simulink library "MedusaPremix"  (R2022b)
settings: Solver=VariableStepAuto  StartTime=0.0  StopTime=10.0  RelTol=1e-3
values from neighbouring files (symbols this model uses):
  PremixConfig = struct('sample_rate_in_hertz', sample_rate_in_hertz,                            'frame_size', frame_size,                            'rgain_SILENT_GAIN', rgain_SILENT_GAIN,                            'granularity', internal_granularity,                            'LR_in', LR_in, 'LR_out', LR_out,                            'CS_in', CS_in, 'CS_out', CS_out,                            'NumCenterOut' ...(+550 chars)    [MedusaPremixInit.m]
  PremixTune = MedusaPremixTuneInit(tuneFileName, headrestTuneFileName, overheadTuneFileName, MedusaParams)    [MedusaPremixInit.m]    (also in MedusaPremixTuneInit.m = load(tuneFileName))
undefined symbols (not defined in the file or in its folder): carModel, mode, MSConfig, Row
libraries: TuneVar x286, TOP x202, dspmtrx3 x146, FeaturePath x86, matrix_library x20, PooliirLib x8, Pooliir x4
(part 17 of 22)

== matlab function MedusaPremix/PremixWithMonoSurroundAndCae/SLC Tuning/Detent Level Right/Trivial Translation ==
  data: TOP output size=[MedusaPremixConfig.LR_out MedusaPremixConfig.LR_in]; detentGain_Right input; MedusaPremixConfig parameter; TOP_CAE output size=[MedusaPremixConfig.LR_out MedusaPremixConfig.NumTailComp.LR]
  events: trigger input FUNCTION_CALL_EVENT
function [TOP, TOP_CAE]  = fcn(detentGain_Right, MedusaPremixConfig)
%#codegen
numLRIn = MedusaPremixConfig.LR_in;
NumCAEWeights = MedusaPremixConfig.NumTailComp.LR;

NumRows = MedusaPremixConfig.LR_out;
NumColumns = numLRIn + NumCAEWeights;
if(~ MedusaPremixConfig.includeCAE)
    NumColumns = numLRIn;
end

% Checks if the parameter satisfies dimensionality requirements
if(detentGain_Right.Size(1) ~= NumRows || detentGain_Right.Size(2) ~= NumColumns)
    TranslateError('The parameter ''medusa_premix_right_detent'' must be a matrix consisting of %d rows and %d columns.', NumRows, NumColumns);
end

% Checks if the parameter values follow bound requirements
checkValues = (detentGain_Right.Value < 0);    
if(sum(sum(checkValues)))       % Results in 0 if all values in the matrix respect the bound requirements
    TranslateError('The weights in ''medusa_premix_right_detent'' must be greater than or equal to 0.');
end

% Assigning the parameter values to respective tuneTOPS
TOP = detentGain_Right.Value(:, 1:numLRIn);
if(~ MedusaPremixConfig.includeCAE)
    TOP_CAE = zeros(NumRows, NumCAEWeights);
else
    TOP_CAE = detentGain_Right.Value(:, numLRIn+1:end);
end

end

== matlab function MedusaPremix/PremixWithMonoSurroundAndCae/SLC Tuning/Interpolation Method/Trivial Translation ==
  data: TOP output; interpolationMethod input
  events: trigger input FUNCTION_CALL_EVENT
function TOP  = fcn(interpolationMethod)
%#codegen
% Checks if the parameter satisfies dimensionality requirements
if(numel(interpolationMethod.Value) ~= 1)
   TranslateError('The parameter ''medusa_surround_db_interpolation'' must be single dimensional.'); 
end

% Checks if the parameter value follows bound requirements
if((interpolationMethod.Value ~= 0) && (interpolationMethod.Value ~= 1))
   TranslateError('The value of ''medusa_surround_db_interpolation'' must be either 0 (for linear interpolation) or 1 (for dB-linear interpolation).'); 
end

TOP = interpolationMethod.Value;

end

== matlab function MedusaPremix/PremixWithMonoSurroundAndCae/SLC Tuning/Max Level CS/Trivial Translation ==
  data: TOP output size=[MedusaPremixConfig.CS_out MedusaPremixConfig.CS_in]; maxGain_CS input; MedusaPremixConfig parameter; TOP_CAE output size=[MedusaPremixConfig.CS_out MedusaPremixConfig.NumTailComp.CS]
  events: trigger input FUNCTION_CALL_EVENT
function [TOP, TOP_CAE] = fcn(maxGain_CS, MedusaPremixConfig)
%#codegen
numCSIn = MedusaPremixConfig.CS_in;
NumCAEWeights = MedusaPremixConfig.NumTailComp.CS;

NumRows = MedusaPremixConfig.CS_out;
NumColumns = numCSIn + NumCAEWeights;
if(~ MedusaPremixConfig.includeCAE)
    NumColumns = numCSIn;
end

% Checks if the parameter satisfies dimensionality requirements
if(maxGain_CS.Size(1) ~= NumRows || maxGain_CS.Size(2) ~= NumColumns)
    TranslateError('The parameter ''medusa_premix_cs_max'' must be a matrix consisting of %d rows and %d columns.', NumRows, NumColumns);
end

% Checks if the parameter values follow bound requirements
checkValues = (maxGain_CS.Value < 0);
if(sum(sum(checkValues)))          % Results in 0 if all values in the matrix respect the bound requirements
    TranslateError('The weights in ''medusa_premix_cs_max'' must be greater than or equal to 0.');
end

% Assigning the parameter values to respective tuneTOPS
TOP = maxGain_CS.Value(:, 1:numCSIn);
if(~ MedusaPremixConfig.includeCAE)
    TOP_CAE = zeros(NumRows, NumCAEWeights);
else
    TOP_CAE = maxGain_CS.Value(:, numCSIn+1:end);
end

end

== matlab function MedusaPremix/PremixWithMonoSurroundAndCae/SLC Tuning/Max Level Left/Trivial Translation ==
  data: TOP output size=[MedusaPremixConfig.LR_out MedusaPremixConfig.LR_in]; maxGain_Left input; MedusaPremixConfig parameter; TOP_CAE output size=[MedusaPremixConfig.LR_out MedusaPremixConfig.NumTailComp.LR]
  events: trigger input FUNCTION_CALL_EVENT
function [TOP, TOP_CAE]  = fcn(maxGain_Left, MedusaPremixConfig)
%#codegen
numLRIn = MedusaPremixConfig.LR_in;
NumCAEWeights = MedusaPremixConfig.NumTailComp.LR;

NumRows = MedusaPremixConfig.LR_out;
NumColumns = numLRIn + NumCAEWeights;
if(~ MedusaPremixConfig.includeCAE)
    NumColumns = numLRIn;
end

% Checks if the parameter satisfies dimensionality requirements
if(maxGain_Left.Size(1) ~= NumRows || maxGain_Left.Size(2) ~= NumColumns)
    TranslateError('The parameter ''medusa_premix_left_max'' must be a matrix consisting of %d rows and %d columns.', NumRows, NumColumns);
end

% Checks if the parameter values follow bound requirements
checkValues = (maxGain_Left.Value < 0);
if(sum(sum(checkValues)))          % Results in 0 if all values in the matrix respect the bound requirements
    TranslateError('The weights in ''medusa_premix_left_max'' must be greater than or equal to 0.');
end

% Assigning the parameter values to respective tuneTOPS
TOP = maxGain_Left.Value(:, 1:numLRIn);
if(~ MedusaPremixConfig.includeCAE)
    TOP_CAE = zeros(NumRows, NumCAEWeights);
else
    TOP_CAE = maxGain_Left.Value(:, numLRIn+1:end);
end

end

== matlab function MedusaPremix/PremixWithMonoSurroundAndCae/SLC Tuning/Max Level Right/Trivial Translation ==
  data: TOP output size=[MedusaPremixConfig.LR_out MedusaPremixConfig.LR_in]; maxGain_Right input; MedusaPremixConfig parameter; TOP_CAE output size=[MedusaPremixConfig.LR_out MedusaPremixConfig.NumTailComp.LR]
  events: trigger input FUNCTION_CALL_EVENT
function [TOP, TOP_CAE]  = fcn(maxGain_Right, MedusaPremixConfig)
%#codegen
numLRIn = MedusaPremixConfig.LR_in;
NumCAEWeights = MedusaPremixConfig.NumTailComp.LR;

NumRows = MedusaPremixConfig.LR_out;
NumColumns = numLRIn + NumCAEWeights;
if(~ MedusaPremixConfig.includeCAE)
    NumColumns = numLRIn;
end

% Checks if the parameter satisfies dimensionality requirements
if(maxGain_Right.Size(1) ~= NumRows || maxGain_Right.Size(2) ~= NumColumns)
    TranslateError('The parameter ''medusa_premix_right_max'' must be a matrix consisting of %d rows and %d columns.', NumRows, NumColumns);
end

% Checks if the parameter values follow bound requirements
checkValues = (maxGain_Right.Value < 0);
if(sum(sum(checkValues)))          % Results in 0 if all values in the matrix respect the bound requirements
    TranslateError('The weights in ''medusa_premix_right_max'' must be greater than or equal to 0.');
end

% Assigning the parameter values to respective tuneTOPS
TOP = maxGain_Right.Value(:, 1:numLRIn);
if(~ MedusaPremixConfig.includeCAE)
    TOP_CAE = zeros(NumRows, NumCAEWeights);
else
    TOP_CAE = maxGain_Right.Value(:, numLRIn+1:end);
end

end

== matlab function MedusaPremix/PremixWithMonoSurroundAndCae/SLC Tuning/Min Level CS/Trivial Translation ==
  data: TOP output size=[MedusaPremixConfig.CS_out MedusaPremixConfig.CS_in]; minGain_CS input; MedusaPremixConfig parameter; TOP_CAE output size=[MedusaPremixConfig.CS_out MedusaPremixConfig.NumTailComp.CS]
  events: trigger input FUNCTION_CALL_EVENT
function [TOP, TOP_CAE]  = fcn(minGain_CS, MedusaPremixConfig)
%#codegen
numCSIn = MedusaPremixConfig.CS_in;
NumCAEWeights = MedusaPremixConfig.NumTailComp.CS;

NumRows = MedusaPremixConfig.CS_out;
NumColumns = numCSIn + NumCAEWeights;
if(~ MedusaPremixConfig.includeCAE)
    NumColumns = numCSIn;
end

% Checks if the parameter satisfies dimensionality requirements
if(minGain_CS.Size(1) ~= NumRows || minGain_CS.Size(2) ~= NumColumns)
    TranslateError('The parameter ''medusa_premix_cs_min'' must be a matrix consisting of %d rows and %d columns.', NumRows, NumColumns);
end

% Checks if the parameter values follow bound requirements
checkValues = (minGain_CS.Value < 0);
if(sum(sum(checkValues)))          % Results in 0 if all values in the matrix respect the bound requirements
    TranslateError('The weights in ''medusa_premix_cs_min'' must be greater than or equal to 0.');
end

% Assigning the parameter values to respective tuneTOPS
TOP = minGain_CS.Value(:, 1:numCSIn);
if(~ MedusaPremixConfig.includeCAE)
    TOP_CAE = zeros(NumRows, NumCAEWeights);
else
    TOP_CAE = minGain_CS.Value(:, numCSIn+1:end);
end

end

== matlab function MedusaPremix/PremixWithMonoSurroundAndCae/SLC Tuning/Min Level Left/Trivial Translation ==
  data: TOP output size=[MedusaPremixConfig.LR_out MedusaPremixConfig.LR_in]; minGain_Left input; MedusaPremixConfig parameter; TOP_CAE output size=[MedusaPremixConfig.LR_out MedusaPremixConfig.NumTailComp.LR]
  events: trigger input FUNCTION_CALL_EVENT
function [TOP, TOP_CAE]  = fcn(minGain_Left, MedusaPremixConfig)
%#codegen
numLRIn = MedusaPremixConfig.LR_in;
NumCAEWeights = MedusaPremixConfig.NumTailComp.LR;

NumRows = MedusaPremixConfig.LR_out;
NumColumns = numLRIn + NumCAEWeights;
if(~ MedusaPremixConfig.includeCAE)
    NumColumns = numLRIn;
end

% Checks if the parameter satisfies dimensionality requirements
if(minGain_Left.Size(1) ~= NumRows || minGain_Left.Size(2) ~= NumColumns)
    TranslateError('The parameter ''medusa_premix_left_min'' must be a matrix consisting of %d rows and %d columns.', NumRows, NumColumns);
end

% Checks if the parameter values follow bound requirements
checkValues = (minGain_Left.Value < 0);
if(sum(sum(checkValues)))          % Results in 0 if all values in the matrix respect the bound requirements
    TranslateError('The weights in ''medusa_premix_left_min'' must be greater than or equal to 0.');
end

% Assigning the parameter values to respective tuneTOPS
TOP = minGain_Left.Value(:, 1:numLRIn);
if(~ MedusaPremixConfig.includeCAE)
    TOP_CAE = zeros(NumRows, NumCAEWeights);
else
    TOP_CAE = minGain_Left.Value(:, numLRIn+1:end);
end

end

== matlab function MedusaPremix/PremixWithMonoSurroundAndCae/SLC Tuning/Min Level Right/Trivial Translation ==
  data: TOP output size=[MedusaPremixConfig.LR_out MedusaPremixConfig.LR_in]; minGain_Right input; MedusaPremixConfig parameter; TOP_CAE output size=[MedusaPremixConfig.LR_out MedusaPremixConfig.NumTailComp.LR]
  events: trigger input FUNCTION_CALL_EVENT
function [TOP, TOP_CAE]  = fcn(minGain_Right, MedusaPremixConfig)
%#codegen
numLRIn = MedusaPremixConfig.LR_in;
NumCAEWeights = MedusaPremixConfig.NumTailComp.LR;

NumRows = MedusaPremixConfig.LR_out;
NumColumns = numLRIn + NumCAEWeights;
if(~ MedusaPremixConfig.includeCAE)
    NumColumns = numLRIn;
end

% Checks if the parameter satisfies dimensionality requirements
if(minGain_Right.Size(1) ~= NumRows || minGain_Right.Size(2) ~= NumColumns)
    TranslateError('The parameter ''medusa_premix_right_min'' must be a matrix consisting of %d rows and %d columns.', NumRows, NumColumns);
end

% Checks if the parameter values follow bound requirements
checkValues = (minGain_Right.Value < 0);
if(sum(sum(checkValues)))          % Results in 0 if all values in the matrix respect the bound requirements
    TranslateError('The weights in ''medusa_premix_right_min'' must be greater than or equal to 0.');
end

% Assigning the parameter values to respective tuneTOPS
TOP = minGain_Right.Value(:, 1:numLRIn);
if(~ MedusaPremixConfig.includeCAE)
    TOP_CAE = zeros(NumRows, NumCAEWeights);
else
    TOP_CAE = minGain_Right.Value(:, numLRIn+1:end);
end

end

== matlab function MedusaPremix/PremixWithMonoSurroundAndCae/Split NTF_check_done ==
  events: fcncall_Left output FUNCTION_CALL_EVENT; trigger input FUNCTION_CALL_EVENT; fcncall_CS output FUNCTION_CALL_EVENT; fcncall_Right output FUNCTION_CALL_EVENT; fcncall_AND output FUNCTION_CALL_EVENT
function FC_Split
% #codegen
% Splits the incoming function call
fcncall_Left();
fcncall_CS();
fcncall_Right();
fcncall_AND();
end

== matlab function MedusaPremix/Premix51WithMonoSurroundAndCae/CS Processing/Mono-Surround/MS Tune/translation ==
  data: phi output; PhaseAngle input; cos_phi output; sin_phi output
  events: trigger input FUNCTION_CALL_EVENT
function [phi, cos_phi, sin_phi]  = fcn(PhaseAngle)
%#codegen
% Checks if the parameter satisfies dimensionality requirements
if(numel(PhaseAngle.Value) ~= 1)
   TranslateError('The parameter ''medusa_mono_c_s_blending_angle_deg'' must be single dimensional.'); 
end

% Checks if the parameter value follows bound requirements
if((PhaseAngle.Value < 0) || (PhaseAngle.Value >= 360))
   TranslateError('The value of ''medusa_mono_c_s_blending_angle_deg'' must be in degrees and can range from 0 to 359.'); 
end

phi = PhaseAngle.Value;
cos_phi = cosd(phi);
sin_phi = sind(phi);

end

== matlab function MedusaPremix/Premix51WithMonoSurroundAndCae/CS Processing/Selective Concatenation ==
  data: COut input; CSOut output; S input; MedusaPremixConfig parameter
function CSOut = fcn(COut, S, MedusaPremixConfig)
%#codegen

% Concatenate monosurround output (if available) to the center outputs
if MedusaPremixConfig.NumSurroundOut==0
    CSOut = COut;
else
    CSOut = [COut S];
end

end

== matlab function MedusaPremix/Premix51WithMonoSurroundAndCae/Fade Inputs/Fade_Trigger_Generation ==
  data: gainDifference input
  events: fadeTrigger_Left output FUNCTION_CALL_EVENT; fadeTrigger_CS output FUNCTION_CALL_EVENT; fadeTrigger_Right output FUNCTION_CALL_EVENT
function Fade_Trigger(gainDifference)
% #codegen
    % Generates function call triggers when incoming fade gain values change
    if(gainDifference > 0)
        fadeTrigger_Left();
        fadeTrigger_CS();
        fadeTrigger_Right();
    end
end

== matlab function MedusaPremix/Premix51WithMonoSurroundAndCae/Fade Tuning/Backward Downmix Max/Trivial Translation ==
  data: TOP output; BackwardDownmixMax input
  events: trigger input FUNCTION_CALL_EVENT
function TOP  = fcn(BackwardDownmixMax)
%#codegen
% Checks if the parameter satisfies dimensionality requirements
if(numel(BackwardDownmixMax.Value) ~= 1)
   TranslateError('The parameter ''medusa_backward_downmix_max'' must be single dimensional.'); 
end

% Checks if the parameter value follows bound requirements
if((BackwardDownmixMax.Value < 0) || (BackwardDownmixMax.Value > 1))
   TranslateError('The value of ''medusa_backward_downmix_max'' must be between 0 and 1.'); 
end

TOP = BackwardDownmixMax.Value;

end

== matlab function MedusaPremix/Premix51WithMonoSurroundAndCae/Fade Tuning/Backward Downmix Threshold/Trivial Translation ==
  data: TOP output; BackwardDownmixThreshold input
  events: trigger input FUNCTION_CALL_EVENT
function TOP  = fcn(BackwardDownmixThreshold)
%#codegen
% Checks if the parameter satisfies dimensionality requirements
if(numel(BackwardDownmixThreshold.Value) ~= 1)
   TranslateError('The parameter ''medusa_backward_downmix_threshold'' must be single dimensional.'); 
end

% Checks if the parameter value follows bound requirements
if((BackwardDownmixThreshold.Value < 0) || (BackwardDownmixThreshold.Value > 1))
   TranslateError('The value of ''medusa_backward_downmix_threshold'' must be between 0 and 1.'); 
end

TOP = BackwardDownmixThreshold.Value;

end

== matlab function MedusaPremix/Premix51WithMonoSurroundAndCae/Fade Tuning/Downmix Weights CS/Trivial Translation ==
  data: TOP output size=[MedusaPremixConfig.CS_out MedusaPremixConfig.CS_in]; downmix_wts_CS input; MedusaPremixConfig parameter; TOP_CAE output size=[MedusaPremixConfig.CS_out MedusaPremixConfig.NumTailComp.CS]
  events: trigger input FUNCTION_CALL_EVENT
function [TOP,TOP_CAE]  = fcn(downmix_wts_CS, MedusaPremixConfig)
%#codegen
numCSIn = MedusaPremixConfig.CS_in;
NumCAEWeights = MedusaPremixConfig.NumTailComp.CS;

NumRows = MedusaPremixConfig.CS_out;
NumColumns = numCSIn + NumCAEWeights;
if(~ MedusaPremixConfig.includeCAE)
    NumColumns = numCSIn;
end

% Checks if the parameter satisfies dimensionality requirements
if(downmix_wts_CS.Size(1) ~= NumRows || downmix_wts_CS.Size(2) ~= NumColumns)
    TranslateError('The parameter ''medusa_premix_downmix_cs'' must be a matrix consisting of %d rows and %d columns.', NumRows, NumColumns);
end

% Checks if the parameter values follow bound requirements
checkValues = (downmix_wts_CS.Value < 0);
if(sum(sum(checkValues)))          % Results in 0 if all values in the matrix respect the bound requirements
    TranslateError('The weights in ''medusa_premix_downmix_CS'' must be greater than or equal to 0.');
end

% Assigning the parameter values to respective tuneTOPS
TOP = downmix_wts_CS.Value(:, 1:numCSIn);
if(~ MedusaPremixConfig.includeCAE)
    TOP_CAE = zeros(NumRows, NumCAEWeights);
else
    TOP_CAE = downmix_wts_CS.Value(:, numCSIn+1:end);
end

end

== matlab function MedusaPremix/Premix/Full Mixing Matrix_Right/Surround Level Control/Ramper/check sequence ==
  data: done output; Premix_currentGain_Right data_store_memory; Premix_targetGain_Right data_store_memory
  events: trigger input FUNCTION_CALL_EVENT
function done = GetCompletedSequence
% #codegen

    global Premix_currentGain_Right;
    global Premix_targetGain_Right;

    % Assume the work is complete until proven otherwise
    done = true;

    for i=1:numel(Premix_targetGain_Right)
       if (Premix_targetGain_Right(i) ~= Premix_currentGain_Right(i))
           done = false; % just proved otherwise
           break;
       end
    end

end

== matlab function MedusaPremix/Premix51WithMonoSurroundAndCae/Fade Tuning/Downmix Weights Left/Trivial Translation ==
  data: TOP output size=[MedusaPremixConfig.LR_out MedusaPremixConfig.LR_in]; downmix_wts_Left input; MedusaPremixConfig parameter; TOP_CAE output size=[MedusaPremixConfig.LR_out MedusaPremixConfig.NumTailComp.LR]
  events: trigger input FUNCTION_CALL_EVENT
function [TOP,TOP_CAE]  = fcn(downmix_wts_Left, MedusaPremixConfig)
%#codegen
numLRIn = MedusaPremixConfig.LR_in;
NumCAEWeights = MedusaPremixConfig.NumTailComp.LR;

NumRows = MedusaPremixConfig.LR_out;
NumColumns = numLRIn + NumCAEWeights;
if(~ MedusaPremixConfig.includeCAE)
    NumColumns = numLRIn;
end

% Checks if the parameter satisfies dimensionality requirements
if(downmix_wts_Left.Size(1) ~= NumRows || downmix_wts_Left.Size(2) ~= NumColumns)
    TranslateError('The parameter ''medusa_premix_downmix_left'' must be a matrix consisting of %d rows and %d columns.', NumRows, NumColumns);
end

% Checks if the parameter values follow bound requirements
checkValues = (downmix_wts_Left.Value < 0);
if(sum(sum(checkValues)))          % Results in 0 if all values in the matrix respect the bound requirements
    TranslateError('The weights in ''medusa_premix_downmix_left'' must be greater than or equal to 0.');
end

% Assigning the parameter values to respective tuneTOPS
TOP = downmix_wts_Left.Value(:, 1:numLRIn);
if(~ MedusaPremixConfig.includeCAE)
    TOP_CAE = zeros(NumRows, NumCAEWeights);
else
    TOP_CAE = downmix_wts_Left.Value(:, numLRIn+1:end);
end

end

== matlab function MedusaPremix/Premix51WithMonoSurroundAndCae/Fade Tuning/Downmix Weights Right/Trivial Translation ==
  data: TOP output size=[MedusaPremixConfig.LR_out MedusaPremixConfig.LR_in]; downmix_wts_Right input; MedusaPremixConfig parameter; TOP_CAE output size=[MedusaPremixConfig.LR_out MedusaPremixConfig.NumTailComp.LR]
  events: trigger input FUNCTION_CALL_EVENT
function [TOP,TOP_CAE]  = fcn(downmix_wts_Right, MedusaPremixConfig)
%#codegen
numLRIn = MedusaPremixConfig.LR_in;
NumCAEWeights = MedusaPremixConfig.NumTailComp.LR;

NumRows = MedusaPremixConfig.LR_out;
NumColumns = numLRIn + NumCAEWeights;
if(~ MedusaPremixConfig.includeCAE)
    NumColumns = numLRIn;
end

% Checks if the parameter satisfies dimensionality requirements
if(downmix_wts_Right.Size(1) ~= NumRows || downmix_wts_Right.Size(2) ~= NumColumns)
    TranslateError('The parameter ''medusa_premix_downmix_right'' must be a matrix consisting of %d rows and %d columns.', NumRows, NumColumns);
end

% Checks if the parameter values follow bound requirements
checkValues = (downmix_wts_Right.Value < 0);
if(sum(sum(checkValues)))          % Results in 0 if all values in the matrix respect the bound requirements
    TranslateError('The weights in ''medusa_premix_downmix_right'' must be greater than or equal to 0.');
end

% Assigning the parameter values to respective tuneTOPS
TOP = downmix_wts_Right.Value(:, 1:numLRIn);
if(~ MedusaPremixConfig.includeCAE)
    TOP_CAE = zeros(NumRows, NumCAEWeights);
else
    TOP_CAE = downmix_wts_Right.Value(:, numLRIn+1:end);
end

end

== matlab function MedusaPremix/Premix51WithMonoSurroundAndCae/Fade Tuning/Forward Downmix Threshold/Trivial Translation ==
  data: TOP output; ForwardDownmixThreshold input
  events: trigger input FUNCTION_CALL_EVENT
function TOP  = fcn(ForwardDownmixThreshold)
%#codegen
% Checks if the parameter satisfies dimensionality requirements
if(numel(ForwardDownmixThreshold.Value) ~= 1)
   TranslateError('The parameter ''medusa_forward_downmix_threshold'' must be single dimensional.'); 
end

% Checks if the parameter value follows bound requirements
if((ForwardDownmixThreshold.Value < 0) || (ForwardDownmixThreshold.Value > 1))
   TranslateError('The value of ''medusa_forward_downmix_threshold'' must be between 0 and 1.'); 
end

TOP = ForwardDownmixThreshold.Value;

end

== matlab function MedusaPremix/Premix51WithMonoSurroundAndCae/Fade Tuning/Foward Downmix Max/Trivial Translation ==
  data: TOP output; ForwardDownmixMax input
  events: trigger input FUNCTION_CALL_EVENT
function TOP  = fcn(ForwardDownmixMax)
%#codegen
% Checks if the parameter satisfies dimensionality requirements
if(numel(ForwardDownmixMax.Value) ~= 1)
   TranslateError('The parameter ''medusa_forward_downmix_max'' must be single dimensional.'); 
end

% Checks if the parameter value follows bound requirements
if((ForwardDownmixMax.Value < 0) || (ForwardDownmixMax.Value > 1))
   TranslateError('The value of ''medusa_forward_downmix_max'' must be between 0 and 1.'); 
end

TOP = ForwardDownmixMax.Value;

end

== matlab function MedusaPremix/Premix51WithMonoSurroundAndCae/Full Mixing Matrix_Center Surround/Fader Downmix/MATLAB Function ==
  data: weights input; weights_CAE input; CAE_Enable input; downmixWeights output; MedusaPremixConfig parameter
function downmixWeights = addCAEGain(weights, weights_CAE, CAE_Enable, MedusaPremixConfig)
% #codegen
    downmixWeights = weights;

    % If CAE is supported and enabled, replace the tail weights with their CAE counterparts
    if(MedusaPremixConfig.includeCAE ==1 && CAE_Enable == 1)
        gainStruct.downmixWeight = weights;  gainStruct.downmixWeight_CAE = weights_CAE;
        gainStructOut = MedusaPremixAddCAEGain(gainStruct, 1, MedusaPremixConfig);
        downmixWeights = gainStructOut.downmixWeight;
    end

end

== matlab function MedusaPremix/Premix51WithMonoSurroundAndCae/Full Mixing Matrix_Center Surround/Surround Level Control/Initialization and RMDL ==
  data: minGain_CS input; minGain_CS_CAE input; detentGain_CS input; detentGain_CS_CAE input; maxGain_CS input; maxGain_CS_CAE input; interpolation_method input; CAE_Enable input; surr_level input; Premix_targetGain_CS data_store_memory; Premix_currentGain_CS data_store_memory; MedusaPremixConfig parameter
  events: trigger input FUNCTION_CALL_EVENT
function Initialization_and_RMDL(minGain_CS, minGain_CS_CAE, detentGain_CS, detentGain_CS_CAE, maxGain_CS, maxGain_CS_CAE, interpolation_method, CAE_Enable, surr_level, MedusaPremixConfig)
% #codegen
    global Premix_currentGain_CS;
    global Premix_targetGain_CS;

    % If CAE is supported and enabled, replace the tail weights with their CAE counterparts
    if(MedusaPremixConfig.includeCAE == 1 && CAE_Enable == 1)
        gainStruct.minGain = minGain_CS;  gainStruct.minGain_CAE = minGain_CS_CAE;
        gainStruct.detentGain = detentGain_CS;  gainStruct.detentGain_CAE = detentGain_CS_CAE;
        gainStruct.maxGain = maxGain_CS;  gainStruct.maxGain_CAE = maxGain_CS_CAE;

        gainStructOut = MedusaPremixAddCAEGain(gainStruct, 1, MedusaPremixConfig);

        minGain_CS = gainStructOut.minGain;
        detentGain_CS = gainStructOut.detentGain;
        maxGain_CS = gainStructOut.maxGain;
    end
    
    % Computing the 'surround' part of mixing gains depending on the surround
    % level index; The other part of mixing gain comes from 'fade downmix'
    gain = MedusaPremixGainComputation(minGain_CS, detentGain_CS, maxGain_CS, interpolation_method, surr_level, MedusaPremixConfig);
    
    % Ramping doesn't take place during RMDL and cold start. Hence, gains
    % are directly pushed to mixing matrix
    Premix_currentGain_CS = gain;
    Premix_targetGain_CS = gain;
end

== matlab function MedusaPremix/Premix51WithMonoSurroundAndCae/Full Mixing Matrix_Center Surround/Surround Level Control/Ramper/check sequence ==
  data: done output; Premix_currentGain_CS data_store_memory; Premix_targetGain_CS data_store_memory
  events: trigger input FUNCTION_CALL_EVENT
function done = GetCompletedSequence
% #codegen

    global Premix_currentGain_CS;
    global Premix_targetGain_CS;

    % Assume the work is complete until proven otherwise
    done = true;

    for i=1:numel(Premix_targetGain_CS)
       if (Premix_targetGain_CS(i) ~= Premix_currentGain_CS(i))
           done = false; % just proved otherwise
           break;
       end
    end

end

== matlab function MedusaPremix/Premix51WithMonoSurroundAndCae/Full Mixing Matrix_Center Surround/Surround Level Control/Ramper/control ==
  data target_gains_linear settings: description=This vector signal must provide a linear target gain for every ramper.
  data: target_gains_linear input; rampRate input; rampTime input; MedusaPremixConfig parameter; Premix_Freeze_CS data_store_memory; Premix_frameCount_CS data_store_memory; Premix_rampCoeff_CS data_store_memory; Premix_targetGain_CS data_store_memory; Premix_currentGain_CS data_store_memory
  events: trigger input FUNCTION_CALL_EVENT
function control(target_gains_linear, rampRate, rampTime, MedusaPremixConfig)
%#codegen

    global Premix_Freeze_CS;
    global Premix_frameCount_CS;
    global Premix_rampCoeff_CS;
    global Premix_targetGain_CS;
    global Premix_currentGain_CS;

    dim_rgain = size(Premix_currentGain_CS);
    rgain_SILENT_GAIN_mat = (MedusaPremixConfig.rgain_SILENT_GAIN)*ones(dim_rgain);

    % Step 1: FREEZE the gain ramper so that we can perform calculations based
    % on the current gain value.
    Premix_Freeze_CS(1) = true; % freeze the gain

    % Step 2: Nudge the gain values a bit if they are sitting at zero.
    % When this control set goes live, ensure that the current gain will move.
    % If current gain is zero, replace with a value very close to zero. What we
    % really want is a value which is on the edge of perception - not too small
    % or large. If the value is too small, we'll waste some of our ramp time
    % in perceived silence. If the value is too large, the audio will lurch
    % into perceptability at the start of the ramp.
    currentgain = max(Premix_currentGain_CS, rgain_SILENT_GAIN_mat);
    targetGain  = max(target_gains_linear, rgain_SILENT_GAIN_mat);
    
    % Step 3a: If a ramp time in milliseconds is provided, ignore the ramp
    % rate in dB/sec (if also provided), otherwise calculate a new ramp time
    % that matches the slope.
    rampTime_ms = single(rampTime)*ones(dim_rgain);
    
    if(~rampTime)
        currentGain_db = 20*log10(currentgain);
        targetGain_db = 20*log10(targetGain);
        diff = abs(currentGain_db - targetGain_db);
        rampTime_ms = diff / single(rampRate) * 1000;
    end
    
    % Step 3b: QUANTIZE the desired ramp time to our FrameSize. Also retrieve 
    % the whole number of frames required to best match requested ramp time.
    % Ensure that at least one frame is used. The frame size will therefore
    % determine the steepest ramp (i.e. within one frame you can go anywhere).
    quantum_ms = 1000 * (MedusaPremixConfig.frame_size) / (MedusaPremixConfig.sample_rate_in_hertz);
    numFrames = rampTime_ms / quantum_ms;
    numFrames = max (1, round(numFrames));

    % In order to have the desired ramp time, the slope must vary dependent
    % on the gain differencebetween target and current value.
    % Ramper's coefficient is therefore calculated as follows:
    %
    %   TargetGain = CurrentGain *( RampCoef ^ (Fs*RampTime_ms/1000) )
    %
    % therefore...
    %
    %                     log(TargetGain/CurrentGain)
    %   log(RampCoef) = ------------------------------
    %                        Fs*(RampTime_ms/1000)
    %
    factor = log( targetGain ./ currentgain );
    RampCoef = exp(factor ./ numFrames);
    
    % Output control signals
    Premix_frameCount_CS  = int32(numFrames);
    Premix_rampCoeff_CS   = single(RampCoef);
    Premix_targetGain_CS  = target_gains_linear;
    Premix_currentGain_CS = currentgain;

    % unfreeze the gain
    Premix_Freeze_CS(1) = false;

end

== matlab function MedusaPremix/Premix/Full Mixing Matrix_Right/Surround Level Control/Ramper/control ==
  data target_gains_linear settings: description=This vector signal must provide a linear target gain for every ramper.
  data: target_gains_linear input; rampRate input; rampTime input; MedusaPremixConfig parameter; Premix_Freeze_Right data_store_memory; Premix_frameCount_Right data_store_memory; Premix_rampCoeff_Right data_store_memory; Premix_targetGain_Right data_store_memory; Premix_currentGain_Right data_store_memory
  events: trigger input FUNCTION_CALL_EVENT
function control(target_gains_linear, rampRate, rampTime, MedusaPremixConfig)
%#codegen

    global Premix_Freeze_Right;
    global Premix_frameCount_Right;
    global Premix_rampCoeff_Right;
    global Premix_targetGain_Right;
    global Premix_currentGain_Right; 

    dim_rgain = size(Premix_currentGain_Right);
    rgain_SILENT_GAIN_mat = (MedusaPremixConfig.rgain_SILENT_GAIN)*ones(dim_rgain);

    % Step 1: FREEZE the gain ramper so that we can perform calculations based
    % on the current gain value.
    Premix_Freeze_Right(1) = true; % freeze the gain

    % Step 2: Nudge the gain values a bit if they are sitting at zero.
    % When this control set goes live, ensure that the current gain will move.
    % If current gain is zero, replace with a value very close to zero. What we
    % really want is a value which is on the edge of perception - not too small
    % or large. If the value is too small, we'll waste some of our ramp time
    % in perceived silence. If the value is too large, the audio will lurch
    % into perceptability at the start of the ramp.
    currentgain = max(Premix_currentGain_Right, rgain_SILENT_GAIN_mat);
    targetGain  = max(target_gains_linear, rgain_SILENT_GAIN_mat);
    
    % Step 3a: If a ramp time in milliseconds is provided, ignore the ramp
    % rate in dB/sec (if also provided), otherwise calculate a new ramp time
    % that matches the slope.
    rampTime_ms = single(rampTime)*ones(dim_rgain);
    
    if(~rampTime)
        currentGain_db = 20*log10(currentgain);
        targetGain_db = 20*log10(targetGain);
        diff = abs(currentGain_db - targetGain_db);
        rampTime_ms = diff / single(rampRate) * 1000;
    end
    
    % Step 3b: QUANTIZE the desired ramp time to our FrameSize. Also retrieve 
    % the whole number of frames required to best match requested ramp time.
    % Ensure that at least one frame is used. The frame size will therefore
    % determine the steepest ramp (i.e. within one frame you can go anywhere).
    quantum_ms = 1000 * (MedusaPremixConfig.frame_size) / (MedusaPremixConfig.sample_rate_in_hertz);
    numFrames = rampTime_ms / quantum_ms;
    numFrames = max (1, round(numFrames));

    % In order to have the desired ramp time, the slope must vary dependent
    % on the gain differencebetween target and current value.
    % Ramper's coefficient is therefore calculated as follows:
    %
    %   TargetGain = CurrentGain *( RampCoef ^ (Fs*RampTime_ms/1000) )
    %
    % therefore...
    %
    %                     log(TargetGain/CurrentGain)
    %   log(RampCoef) = ------------------------------
    %                        Fs*(RampTime_ms/1000)
    %
    factor = log( targetGain ./ currentgain );
    RampCoef = exp(factor ./ numFrames);
    
    % Output control signals
    Premix_frameCount_Right  = int32(numFrames);
    Premix_rampCoeff_Right   = single(RampCoef);
    Premix_targetGain_Right  = target_gains_linear;
    Premix_currentGain_Right = currentgain;

    % unfreeze the gain
    Premix_Freeze_Right(1) = false;

end

== matlab function MedusaPremix/Premix51WithMonoSurroundAndCae/Full Mixing Matrix_Center Surround/Surround Level Control/Ramper/process ==
  data: Premix_Freeze_CS data_store_memory; Premix_currentGain_CS data_store_memory; Premix_targetGain_CS data_store_memory; Premix_frameCount_CS data_store_memory; Premix_rampCoeff_CS data_store_memory
function process
%#codegen

    global Premix_Freeze_CS;
    global Premix_currentGain_CS;
    global Premix_targetGain_CS;
    global Premix_frameCount_CS;
    global Premix_rampCoeff_CS;

    for i = 1:numel(Premix_currentGain_CS)
        if (Premix_Freeze_CS(1) == false)
            if (Premix_frameCount_CS(i) == 0)
                % The ramp is finished. Stop ramping and SNAP to the target
                Premix_currentGain_CS(i) = Premix_targetGain_CS(i);
            else
                % The ramp is *NOT* frozen or done: gain is moving
                Premix_currentGain_CS(i) = Premix_currentGain_CS(i)*Premix_rampCoeff_CS(i);
                Premix_frameCount_CS(i) = Premix_frameCount_CS(i) - 1;
            end
        end
    end
    
end

== matlab function MedusaPremix/Premix51WithMonoSurroundAndCae/Full Mixing Matrix_Center Surround/Surround Level Control/Target Gain Computation ==
  data: minGain_CS input; minGain_CS_CAE input; detentGain_CS input; detentGain_CS_CAE input; maxGain_CS input; maxGain_CS_CAE input; interpolation_method input; CAE_Enable input; surr_level input; gain_out output; MedusaPremixConfig parameter
  events: trigger input FUNCTION_CALL_EVENT
function gain_out = generate_gain(minGain_CS, minGain_CS_CAE, detentGain_CS, detentGain_CS_CAE, maxGain_CS, maxGain_CS_CAE, interpolation_method, CAE_Enable, surr_level, MedusaPremixConfig)
% #codegen

    % If CAE is supported and enabled, replace the tail weights with their CAE counterparts
    if(MedusaPremixConfig.includeCAE == 1 && CAE_Enable == 1)
        gainStruct.minGain = minGain_CS;  gainStruct.minGain_CAE = minGain_CS_CAE;
        gainStruct.detentGain = detentGain_CS;  gainStruct.detentGain_CAE = detentGain_CS_CAE;
        gainStruct.maxGain = maxGain_CS;  gainStruct.maxGain_CAE = maxGain_CS_CAE;

        gainStructOut = MedusaPremixAddCAEGain(gainStruct, 1, MedusaPremixConfig);

        minGain_CS = gainStructOut.minGain;
        detentGain_CS = gainStructOut.detentGain;
        maxGain_CS = gainStructOut.maxGain;
    end

    % Computing the 'surround' part of mixing gains depending on the surround
    % level index; The other part of mixing gain comes from 'fade downmix'
    targetGain = MedusaPremixGainComputation(minGain_CS, detentGain_CS, maxGain_CS, interpolation_method, surr_level, MedusaPremixConfig);
    
    gain_out = targetGain;
end

== matlab function MedusaPremix/Premix51WithMonoSurroundAndCae/Full Mixing Matrix_Left/Fader Downmix/MATLAB Function ==
  data: weights input; weights_CAE input; CAE_Enable input; downmixWeights output; MedusaPremixConfig parameter
function downmixWeights = addCAEGain(weights, weights_CAE, CAE_Enable, MedusaPremixConfig)
% #codegen
    downmixWeights = weights;
    
    % If CAE is supported and enabled, replace the tail weights with their CAE counterparts
    if(MedusaPremixConfig.includeCAE == 1 && CAE_Enable == 1)
        gainStruct.downmixWeight = weights;  gainStruct.downmixWeight_CAE = weights_CAE;
        gainStructOut = MedusaPremixAddCAEGain(gainStruct, 0, MedusaPremixConfig);
        downmixWeights = gainStructOut.downmixWeight;
    end

end

== matlab function MedusaPremix/Premix51WithMonoSurroundAndCae/Full Mixing Matrix_Left/Surround Level Control/Initialization and RMDL ==
  data: minGain_Left input; minGain_Left_CAE input; detentGain_Left input; detentGain_Left_CAE input; maxGain_Left input; maxGain_Left_CAE input; interpolation_method input; CAE_Enable input; surr_level input; MedusaPremixConfig parameter; Premix_currentGain_Left data_store_memory; Premix_targetGain_Left data_store_memory
  events: trigger input FUNCTION_CALL_EVENT
function generate_gain(minGain_Left, minGain_Left_CAE, detentGain_Left, detentGain_Left_CAE, maxGain_Left, maxGain_Left_CAE, interpolation_method, CAE_Enable, surr_level, MedusaPremixConfig)
% #codegen
    global Premix_currentGain_Left;
    global Premix_targetGain_Left;

    % If CAE is supported and enabled, replace the tail weights with their CAE counterparts
    if(MedusaPremixConfig.includeCAE == 1 && CAE_Enable == 1)
        gainStruct.minGain = minGain_Left;  gainStruct.minGain_CAE = minGain_Left_CAE;
        gainStruct.detentGain = detentGain_Left;  gainStruct.detentGain_CAE = detentGain_Left_CAE;
        gainStruct.maxGain = maxGain_Left;  gainStruct.maxGain_CAE = maxGain_Left_CAE;

        gainStructOut = MedusaPremixAddCAEGain(gainStruct, 0, MedusaPremixConfig);

        minGain_Left = gainStructOut.minGain;
        detentGain_Left = gainStructOut.detentGain;
        maxGain_Left = gainStructOut.maxGain;
    end
    
    % Computing the 'surround' part of mixing gains depending on the surround
    % level index; The other part of mixing gain comes from 'fade downmix'
    gain = MedusaPremixGainComputation(minGain_Left, detentGain_Left, maxGain_Left, interpolation_method, surr_level, MedusaPremixConfig);

    % Ramping doesn't take place during RMDL and cold start. Hence, gains
    % are directly pushed to mixing matrix
    Premix_currentGain_Left = gain;
    Premix_targetGain_Left = gain;

end

== matlab function MedusaPremix/Premix51WithMonoSurroundAndCae/Full Mixing Matrix_Left/Surround Level Control/Ramper/check sequence ==
  data: done output; Premix_currentGain_Left data_store_memory; Premix_targetGain_Left data_store_memory
  events: trigger input FUNCTION_CALL_EVENT
function done = GetCompletedSequence
% #codegen

    global Premix_currentGain_Left;
    global Premix_targetGain_Left;

    % Assume the work is complete until proven otherwise
    done = true;

    for i=1:numel(Premix_targetGain_Left)
       if (Premix_targetGain_Left(i) ~= Premix_currentGain_Left(i))
           done = false; % just proved otherwise
           break;
       end
    end

end

== matlab function MedusaPremix/Premix51WithMonoSurroundAndCae/Full Mixing Matrix_Left/Surround Level Control/Ramper/control ==
  data target_gains_linear settings: description=This vector signal must provide a linear target gain for every ramper.
  data: target_gains_linear input; rampRate input; rampTime input; MedusaPremixConfig parameter; Premix_Freeze_Left data_store_memory; Premix_frameCount_Left data_store_memory; Premix_rampCoeff_Left data_store_memory; Premix_targetGain_Left data_store_memory; Premix_currentGain_Left data_store_memory
  events: trigger input FUNCTION_CALL_EVENT
function control(target_gains_linear, rampRate, rampTime, MedusaPremixConfig)
%#codegen

    global Premix_Freeze_Left;
    global Premix_frameCount_Left;
    global Premix_rampCoeff_Left;
    global Premix_targetGain_Left;
    global Premix_currentGain_Left;  

    dim_rgain = size(Premix_currentGain_Left);
    rgain_SILENT_GAIN_mat = (MedusaPremixConfig.rgain_SILENT_GAIN)*ones(dim_rgain);

    % Step 1: FREEZE the gain ramper so that we can perform calculations based
    % on the current gain value.
    Premix_Freeze_Left(1) = true; % freeze the gain

    % Step 2: Nudge the gain values a bit if they are sitting at zero.
    % When this control set goes live, ensure that the current gain will move.
    % If current gain is zero, replace with a value very close to zero. What we
    % really want is a value which is on the edge of perception - not too small
    % or large. If the value is too small, we'll waste some of our ramp time
    % in perceived silence. If the value is too large, the audio will lurch
    % into perceptability at the start of the ramp.
    currentgain = max(Premix_currentGain_Left, rgain_SILENT_GAIN_mat);
    targetGain  = max(target_gains_linear, rgain_SILENT_GAIN_mat);
    
    % Step 3a: If a ramp time in milliseconds is provided, ignore the ramp
    % rate in dB/sec (if also provided), otherwise calculate a new ramp time
    % that matches the slope.
    rampTime_ms = single(rampTime)*ones(dim_rgain);
    
    if(~rampTime)
        currentGain_db = 20*log10(currentgain);
        targetGain_db = 20*log10(targetGain);
        diff = abs(currentGain_db - targetGain_db);
        rampTime_ms = diff / single(rampRate) * 1000;
    end
    
    % Step 3b: QUANTIZE the desired ramp time to our FrameSize. Also retrieve 
    % the whole number of frames required to best match requested ramp time.
    % Ensure that at least one frame is used. The frame size will therefore
    % determine the steepest ramp (i.e. within one frame you can go anywhere).
    quantum_ms = 1000 * (MedusaPremixConfig.frame_size) / (MedusaPremixConfig.sample_rate_in_hertz);
    numFrames = rampTime_ms / quantum_ms;
    numFrames = max (1, round(numFrames));

    % In order to have the desired ramp time, the slope must vary dependent
    % on the gain differencebetween target and current value.
    % Ramper's coefficient is therefore calculated as follows:
    %
    %   TargetGain = CurrentGain *( RampCoef ^ (Fs*RampTime_ms/1000) )
    %
    % therefore...
    %
    %                     log(TargetGain/CurrentGain)
    %   log(RampCoef) = ------------------------------
    %                        Fs*(RampTime_ms/1000)
    %
    factor = log( targetGain ./ currentgain );
    RampCoef = exp(factor ./ numFrames);

    % Output control signals
    Premix_frameCount_Left  = int32(numFrames);
    Premix_rampCoeff_Left   = single(RampCoef);
    Premix_targetGain_Left  = target_gains_linear;
    Premix_currentGain_Left = currentgain;

    % unfreeze the gain
    Premix_Freeze_Left(1) = false;

end

== matlab function MedusaPremix/Premix51WithMonoSurroundAndCae/Full Mixing Matrix_Left/Surround Level Control/Ramper/process ==
  data: Premix_Freeze_Left data_store_memory; Premix_currentGain_Left data_store_memory; Premix_targetGain_Left data_store_memory; Premix_frameCount_Left data_store_memory; Premix_rampCoeff_Left data_store_memory
function process
%#codegen

    global Premix_Freeze_Left;
    global Premix_currentGain_Left;
    global Premix_targetGain_Left;
    global Premix_frameCount_Left;
    global Premix_rampCoeff_Left;

    for i = 1:numel(Premix_currentGain_Left)
        if (Premix_Freeze_Left(1) == false)
            if (Premix_frameCount_Left(i) == 0)
                % The ramp is finished. Stop ramping and SNAP to the target
                Premix_currentGain_Left(i) = Premix_targetGain_Left(i);
            else
                % The ramp is *NOT* frozen or done: gain is moving
                Premix_currentGain_Left(i) = Premix_currentGain_Left(i)*Premix_rampCoeff_Left(i);
                Premix_frameCount_Left(i) = Premix_frameCount_Left(i) - 1;
            end
        end
    end
    
end

== matlab function MedusaPremix/Premix51WithMonoSurroundAndCae/Full Mixing Matrix_Left/Surround Level Control/Target Gain Computation ==
  data: minGain_Left input; minGain_Left_CAE input; detentGain_Left input; detentGain_Left_CAE input; maxGain_Left input; maxGain_Left_CAE input; interpolation_method input; CAE_Enable input; surr_level input; gain_out output; MedusaPremixConfig parameter
  events: trigger input FUNCTION_CALL_EVENT
function gain_out = generate_gain(minGain_Left, minGain_Left_CAE, detentGain_Left, detentGain_Left_CAE, maxGain_Left, maxGain_Left_CAE, interpolation_method, CAE_Enable, surr_level, MedusaPremixConfig)
% #codegen

    % If CAE is supported and enabled, replace the tail weights with their CAE counterparts
    if(MedusaPremixConfig.includeCAE == 1 && CAE_Enable == 1)
        gainStruct.minGain = minGain_Left;  gainStruct.minGain_CAE = minGain_Left_CAE;
        gainStruct.detentGain = detentGain_Left;  gainStruct.detentGain_CAE = detentGain_Left_CAE;
        gainStruct.maxGain = maxGain_Left;  gainStruct.maxGain_CAE = maxGain_Left_CAE;

        gainStructOut = MedusaPremixAddCAEGain(gainStruct, 0, MedusaPremixConfig);

        minGain_Left = gainStructOut.minGain;
        detentGain_Left = gainStructOut.detentGain;
        maxGain_Left = gainStructOut.maxGain;
    end

    % Computing the 'surround' part of mixing gains depending on the surround
    % level index; The other part of mixing gain comes from 'fade downmix'
    targetGain = MedusaPremixGainComputation(minGain_Left, detentGain_Left, maxGain_Left, interpolation_method, surr_level, MedusaPremixConfig);
    
    gain_out = targetGain;
end

== matlab function MedusaPremix/Premix51WithMonoSurroundAndCae/Full Mixing Matrix_Right/Fader Downmix/MATLAB Function ==
  data: weights input; weights_CAE input; CAE_Enable input; downmixWeights output; MedusaPremixConfig parameter
function downmixWeights = addCAEGain(weights, weights_CAE, CAE_Enable, MedusaPremixConfig)
% #codegen
    downmixWeights = weights;
    
    % If CAE is supported and enabled, replace the tail weights with their CAE counterparts
    if(MedusaPremixConfig.includeCAE == 1 && CAE_Enable == 1)
        gainStruct.downmixWeight = weights;  gainStruct.downmixWeight_CAE = weights_CAE;
        gainStructOut = MedusaPremixAddCAEGain(gainStruct, 0, MedusaPremixConfig);
        downmixWeights = gainStructOut.downmixWeight;
    end
    
end

== matlab function MedusaPremix/Premix51WithMonoSurroundAndCae/Full Mixing Matrix_Right/Surround Level Control/Initialization and RMDL ==
  data: minGain_Right input; minGain_Right_CAE input; detentGain_Right input; detentGain_Right_CAE input; maxGain_Right input; maxGain_Right_CAE input; interpolation_method input; CAE_Enable input; surr_level input; MedusaPremixConfig parameter; Premix_currentGain_Right data_store_memory; Premix_targetGain_Right data_store_memory
  events: trigger input FUNCTION_CALL_EVENT
function generate_gain(minGain_Right, minGain_Right_CAE, detentGain_Right, detentGain_Right_CAE, maxGain_Right, maxGain_Right_CAE, interpolation_method, CAE_Enable, surr_level, MedusaPremixConfig)
% #codegen
    global Premix_currentGain_Right;
    global Premix_targetGain_Right;
    
    % If CAE is supported and enabled, replace the tail weights with their CAE counterparts
    if(MedusaPremixConfig.includeCAE == 1 && CAE_Enable == 1)
        gainStruct.minGain = minGain_Right;  gainStruct.minGain_CAE = minGain_Right_CAE;
        gainStruct.detentGain = detentGain_Right;  gainStruct.detentGain_CAE = detentGain_Right_CAE;
        gainStruct.maxGain = maxGain_Right;  gainStruct.maxGain_CAE = maxGain_Right_CAE;

        gainStructOut = MedusaPremixAddCAEGain(gainStruct, 0, MedusaPremixConfig);

        minGain_Right = gainStructOut.minGain;
        detentGain_Right = gainStructOut.detentGain;
        maxGain_Right = gainStructOut.maxGain;
    end
    
    % Computing the 'surround' part of mixing gains depending on the surround
    % level index; The other part of mixing gain comes from 'fade downmix'
    gain = MedusaPremixGainComputation(minGain_Right, detentGain_Right, maxGain_Right, interpolation_method, surr_level, MedusaPremixConfig);
    
    % Ramping doesn't take place during RMDL and cold start. Hence, gains
    % are directly pushed to mixing matrix
    Premix_currentGain_Right = gain;
    Premix_targetGain_Right = gain;
end

== matlab function MedusaPremix/Premix51WithMonoSurroundAndCae/Full Mixing Matrix_Right/Surround Level Control/Ramper/check sequence ==
  data: done output; Premix_currentGain_Right data_store_memory; Premix_targetGain_Right data_store_memory
  events: trigger input FUNCTION_CALL_EVENT
function done = GetCompletedSequence
% #codegen

    global Premix_currentGain_Right;
    global Premix_targetGain_Right;

    % Assume the work is complete until proven otherwise
    done = true;

    for i=1:numel(Premix_targetGain_Right)
       if (Premix_targetGain_Right(i) ~= Premix_currentGain_Right(i))
           done = false; % just proved otherwise
           break;
       end
    end

end
